simulink model "Reversal_voltage"  (R2020a)
settings: Solver=VariableStepAuto  StartTime=0.0  StopTime=10.0  RelTol=1e-3
settings Model: Creator=shushushu  LastModifiedBy=shushushu

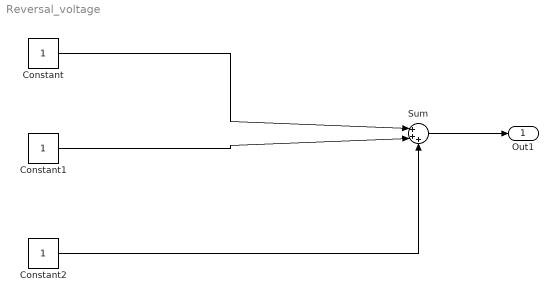
== system Reversal_voltage ==
  Constant : Constant
  Constant1 : Constant
  Constant2 : Constant
  Sum : Sum  Inputs=|+++
  Out1 : Outport
  wires:
  Constant/1 -> Sum/1
  Constant1/1 -> Sum/2
  Constant2/1 -> Sum/3
  Sum/1 -> Out1/1
